simulink model "Final_Project_Pt5"  (R2024a)
settings: Solver=VariableStepAuto  StartTime=0.0  StopTime=tspan  FixedStep=10  RelTol=1e-3
values from neighbouring files (symbols this model uses):
  E_b_ECI_0 = C2EulerAngles(C_b_ECI_0)    [A421_FinalProject_Pt5.m]    (also in A421_FinalProject_Pt6.m; Final_Project_Part_3_disturbances.m; Final_Project_Part_3_disturbances_init_Template-1.m; Final_Project_Part_3_disturbances_init_Template.m)
  epsilon_b_ECI_0 = [-.2; .4; .2]    [A421_FinalProject_Pt6.m]    (also in hw5.m)
  J = [812.04 0 0; 0 545.37 0; 0 0 627.71]    [A421_FinalProject_Pt5.m]    (also in A421_FinalProject_Pt6.m; Final_Project_Part_3_disturbances_torques.m; Final_Project_Pt4.m; hw5.m = diag([1200, 2000, 2800]))
  JD_0 = 2460390    [A421_FinalProject_Pt5.m]    (also in A421_FinalProject_Pt6.m; Final_Project_Part_3_disturbances.m; Final_Project_Part_3_disturbances_init_Template-1.m; Final_Project_Part_3_disturbances_init_Template.m)
  Kd = J*2*zeta*wn*[1;1;1]    [A421_FinalProject_Pt5.m]    (also in A421_FinalProject_Pt6.m = J*2*zeta*wn; hw5.m = J*2*zeta*wn.*eye(3))
  Kp = 2*J*wn^2*[1;1;1]    [A421_FinalProject_Pt5.m]    (also in A421_FinalProject_Pt6.m = 2*J*wn^2.; hw5.m = 2*J*wn^2*eye(3))
  m_b = [0;0;-0.5]    [A421_FinalProject_Pt5.m]    (also in A421_FinalProject_Pt6.m; Final_Project_Pt4.m)
  q_b_ECI_0 = C2quat(C_b_ECI_0)    [A421_FinalProject_Pt5.m]    (also in A421_FinalProject_Pt6.m = [epsilon_b_ECI_0; sqrt(1-norm(epsilon_b_ECI_0)^2)]; Final_Project_Part_3_disturbances.m; Final_Project_Part_3_disturbances_init_Template-1.m; Final_Project_Part_3_disturbances_init_Template.m)
  q_C = [epsilon_C; sqrt(1-norm(epsilon_C)^2)]    [A421_FinalProject_Pt6.m]    (also in hw5.m)
  r_ECI_0 = rECI    [A421_FinalProject_Pt5.m]    (also in A421_FinalProject_Pt6.m; Final_Project_Pt4.m)
  sun_ECI = [1;0;0]    [A421_FinalProject_Pt5.m]    (also in A421_FinalProject_Pt6.m; Final_Project_Part_3_disturbances_torques.m; Final_Project_Pt4.m)
  surfaceProperties = [Areas_1 cps_1 normals_1; Areas_2 cps_2 normals_2; Areas_3 cps_3 normals_3; Areas_4 cps_4 normals_4]    [A421_FinalProject_Pt5.m]    (also in A421_FinalProject_Pt6.m; Final_Project_Part_3_disturbances.m = [Areas cps normals]; Final_Project_Part_3_disturbances_init_Template-1.m = [Areas cps normals]; Final_Project_Part_3_disturbances_init_Template.m = [Areas cps normals])
  T = [0;0;0]    [A421_FinalProject_Pt6.m]    (also in hw5.m; main.m)
  v_ECI_0 = vECI    [A421_FinalProject_Pt5.m]    (also in A421_FinalProject_Pt6.m; Final_Project_Pt4.m)
  w_b_ECI_0 = [0.001; -0.001; 0.002]    [A421_FinalProject_Pt5.m]    (also in A421_FinalProject_Pt6.m; Final_Project_Part_3_disturbances.m; Final_Project_Part_3_disturbances_init_Template-1.m; Final_Project_Part_3_disturbances_init_Template.m)
settings Model: Creator=emehiel  LastModifiedBy=Jacob
settings SolverCC: AlgebraicLoopSolver=TrustRegion
settings OptimizationCC: ReuseModelBlockBuffer=off
settings DebuggingCC: UnconnectedInputMsg=warning  UnconnectedOutputMsg=warning  UnconnectedLineMsg=warning
settings ModelReferenceCC: EnableRefExpFcnMdlSchedulingChecks=on
settings RTWCC: GPUComputeCapability=3.5

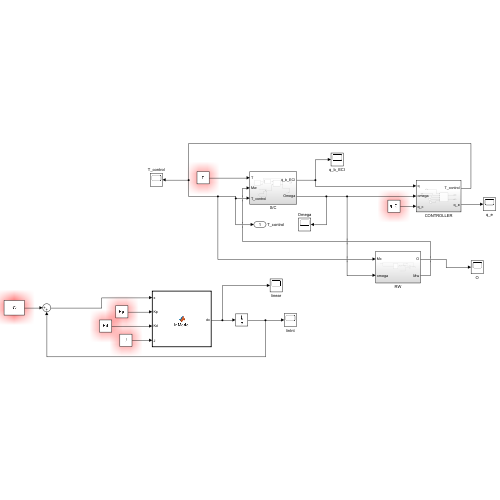
[thumbnail: Simulink's stored preview of the top-level diagram]
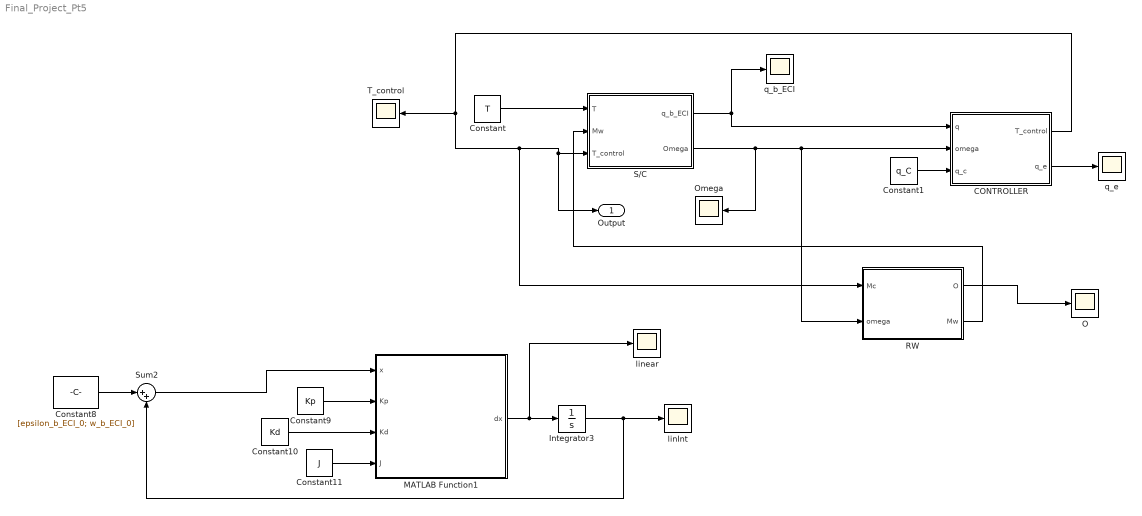
== system Final_Project_Pt5 ==
  CONTROLLER : Subsystem
  Constant : Constant  Value=T  VectorParams1D=off
  Constant1 : Constant  Value=q_C
  Constant10 : Constant  Value=Kd
  Constant11 : Constant  Value=J
  Constant8 : Constant  Value=[epsilon_b_ECI_0; w_b_ECI_0]
  Constant9 : Constant  Value=Kp
  Integrator3 : Integrator
  MATLAB Function1 : MATLAB Function  TreatAsAtomicUnit=on
  O : Scope
  Omega : Scope
  RW : Subsystem
  S/C : Subsystem
  Sum2 : Sum  Inputs=|++
  T_control : Scope
  linInt : Scope
  linear : Scope
  q_b_ECI : Scope
  q_e : Scope
  Output : Outport  SignalName=T_control
  wires:
  Constant/1 -> S/C/1(T)
  CONTROLLER/1(T_control) -> RW/1(Mc), Output/1, S/C/3(T_control), T_control/1
  S/C/2(Omega) -> RW/2(omega), CONTROLLER/2(omega), Omega/1
  CONTROLLER/2(q_e) -> q_e/1
  Constant1/1 -> CONTROLLER/3(q_c)
  Constant11/1 -> MATLAB Function1/4(J)
  Constant10/1 -> MATLAB Function1/3(Kd)
  Constant9/1 -> MATLAB Function1/2(Kp)
  MATLAB Function1/1(dx) -> linear/1, Integrator3/1
  Constant8/1 -> Sum2/1
  Sum2/1 -> MATLAB Function1/1(x)
  Integrator3/1 -> Sum2/2, linInt/1
  S/C/1(q_b_ECI) -> q_b_ECI/1, CONTROLLER/1(q)
  RW/1(O) -> O/1
  RW/2(Mw) -> S/C/2(Mw)

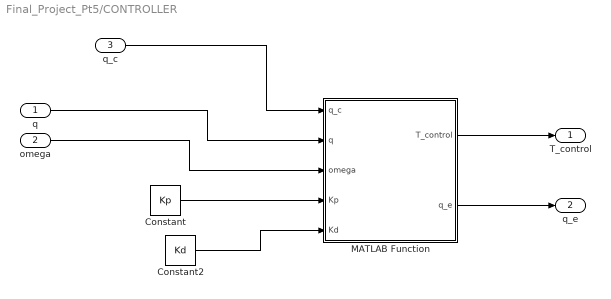
== system Final_Project_Pt5/CONTROLLER ==
  q : Inport
  omega : Inport  Port=2
  q_c : Inport  Port=3
  Constant : Constant  Value=Kp
  Constant2 : Constant  Value=Kd
  MATLAB Function : MATLAB Function  TreatAsAtomicUnit=on
  T_control : Outport
  q_e : Outport  Port=2
  wires:
  q/1 -> MATLAB Function/2(q)
  omega/1 -> MATLAB Function/3(omega)
  Constant/1 -> MATLAB Function/4(Kp)
  Constant2/1 -> MATLAB Function/5(Kd)
  MATLAB Function/2(q_e) -> q_e/1
  q_c/1 -> MATLAB Function/1(q_c)
  MATLAB Function/1(T_control) -> T_control/1

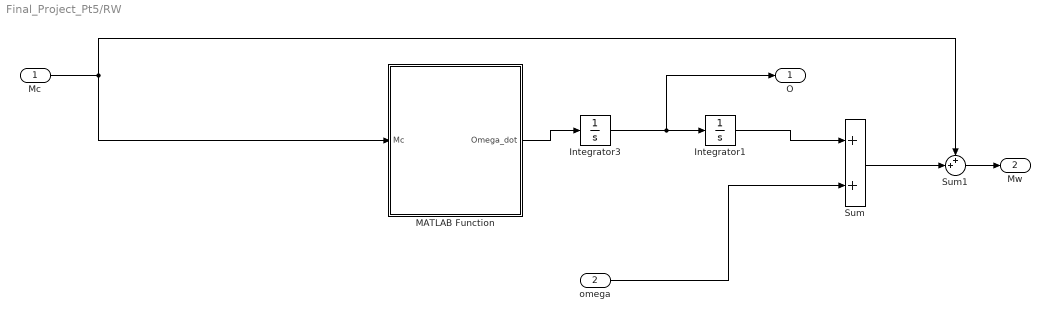
== system Final_Project_Pt5/RW ==
  Mc : Inport
  omega : Inport  Port=2
  Integrator1 : Integrator
  Integrator3 : Integrator
  MATLAB Function : MATLAB Function  TreatAsAtomicUnit=on
  Sum : Sum
  Sum1 : Sum  Inputs=++|
  O : Outport
  Mw : Outport  Port=2
  wires:
  omega/1 -> Sum/2
  Integrator3/1 -> Integrator1/1, O/1
  MATLAB Function/1(Omega_dot) -> Integrator3/1
  Integrator1/1 -> Sum/1
  Sum/1 -> Sum1/2
  Mc/1 -> MATLAB Function/1(Mc), Sum1/1
  Sum1/1 -> Mw/1

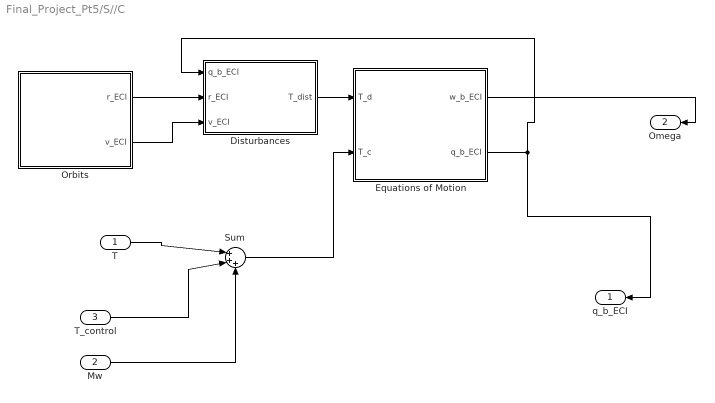
== system Final_Project_Pt5/S//C ==
  T : Inport
  Mw : Inport  Port=2
  T_control : Inport  Port=3
  Disturbances : Subsystem
  Equations of Motion : Subsystem
  Orbits : Subsystem
  Sum : Sum  Inputs=|+++
  q_b_ECI : Outport
  Omega : Outport  Port=2
  wires:
  T/1 -> Sum/1
  T_control/1 -> Sum/2
  Orbits/1(r_ECI) -> Disturbances/2(r_ECI)
  Disturbances/1(T_dist) -> Equations of Motion/1(T_d)
  Orbits/2(v_ECI) -> Disturbances/3(v_ECI)
  Equations of Motion/1(w_b_ECI) -> Omega/1
  Sum/1 -> Equations of Motion/2(T_c)
  Equations of Motion/2(q_b_ECI) -> Disturbances/1(q_b_ECI), q_b_ECI/1
  Mw/1 -> Sum/3

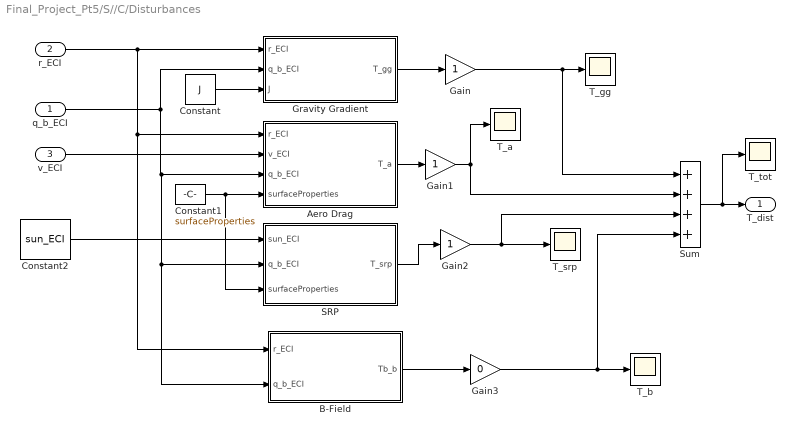
== system Final_Project_Pt5/S//C/Disturbances ==
  q_b_ECI : Inport
  r_ECI : Inport  Port=2
  v_ECI : Inport  Port=3
  Aero Drag : MATLAB Function  TreatAsAtomicUnit=on
  B-Field : Subsystem
  Constant : Constant  Value=J
  Constant1 : Constant  Value=surfaceProperties
  Constant2 : Constant  Value=sun_ECI
  Gain : Gain
  Gain1 : Gain
  Gain2 : Gain
  Gain3 : Gain  Gain=0
  Gravity Gradient : MATLAB Function  TreatAsAtomicUnit=on
  SRP : MATLAB Function  TreatAsAtomicUnit=on
  Sum : Sum  Inputs=++++
  T_a : Scope
  T_b : Scope
  T_gg : Scope
  T_srp : Scope
  T_tot : Scope
  T_dist : Outport
  wires:
  Sum/1 -> T_tot/1, T_dist/1
  Constant1/1 -> SRP/3(surfaceProperties), Aero Drag/4(surfaceProperties)
  v_ECI/1 -> Aero Drag/2(v_ECI)
  q_b_ECI/1 -> B-Field/2(q_b_ECI), SRP/2(q_b_ECI), Aero Drag/3(q_b_ECI), Gravity Gradient/2(q_b_ECI)
  Constant/1 -> Gravity Gradient/3(J)
  Constant2/1 -> SRP/1(sun_ECI)
  r_ECI/1 -> B-Field/1(r_ECI), Aero Drag/1(r_ECI), Gravity Gradient/1(r_ECI)
  Gain/1 -> Sum/1, T_gg/1
  Gain1/1 -> Sum/2, T_a/1
  Gain2/1 -> Sum/3, T_srp/1
  Gain3/1 -> T_b/1, Sum/4
  B-Field/1(Tb_b) -> Gain3/1
  Gravity Gradient/1(T_gg) -> Gain/1
  Aero Drag/1(T_a) -> Gain1/1
  SRP/1(T_srp) -> Gain2/1

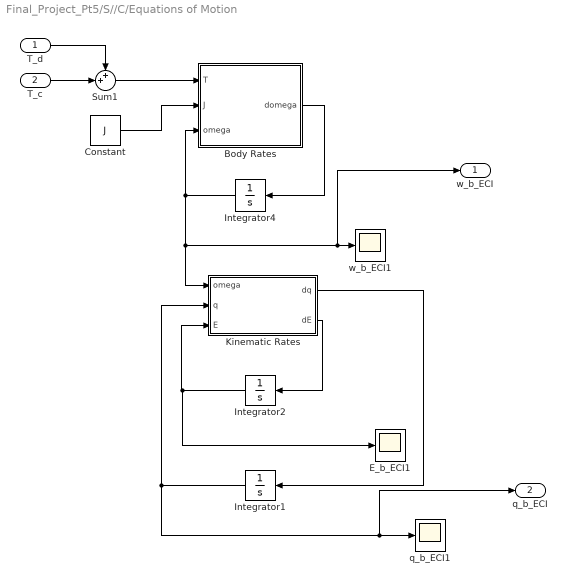
== system Final_Project_Pt5/S//C/Equations of Motion ==
  T_d : Inport
  T_c : Inport  Port=2
  Body Rates : MATLAB Function  TreatAsAtomicUnit=on
  Constant : Constant  Value=J
  E_b_ECI1 : Scope
  Integrator1 : Integrator  InitialCondition=q_b_ECI_0
  Integrator2 : Integrator  InitialCondition=E_b_ECI_0
  Integrator4 : Integrator  InitialCondition=w_b_ECI_0
  Kinematic Rates : MATLAB Function  TreatAsAtomicUnit=on
  Sum1 : Sum  Inputs=++|
  q_b_ECI1 : Scope
  w_b_ECI1 : Scope
  w_b_ECI : Outport  VectorParamsAs1DForOutWhenUnconnected=off
  q_b_ECI : Outport  Port=2  VectorParamsAs1DForOutWhenUnconnected=off
  wires:
  Integrator2/1 -> E_b_ECI1/1, Kinematic Rates/3(E)
  Sum1/1 -> Body Rates/1(T)
  Constant/1 -> Body Rates/2(J)
  T_d/1 -> Sum1/1
  T_c/1 -> Sum1/2
  Integrator1/1 -> q_b_ECI/1, q_b_ECI1/1, Kinematic Rates/2(q)
  Integrator4/1 -> Body Rates/3(omega), w_b_ECI/1, w_b_ECI1/1, Kinematic Rates/1(omega)
  Kinematic Rates/1(dq) -> Integrator1/1
  Kinematic Rates/2(dE) -> Integrator2/1
  Body Rates/1(domega) -> Integrator4/1

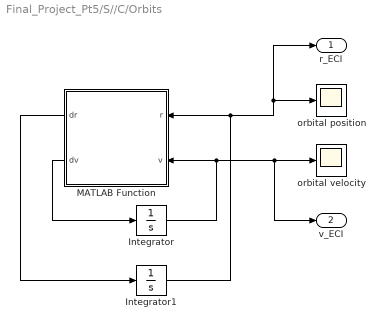
== system Final_Project_Pt5/S//C/Orbits ==
  Integrator : Integrator  InitialCondition=v_ECI_0
  Integrator1 : Integrator  InitialCondition=r_ECI_0
  MATLAB Function : MATLAB Function  TreatAsAtomicUnit=on
  orbital position : Scope
  orbital velocity : Scope
  r_ECI : Outport  VectorParamsAs1DForOutWhenUnconnected=off
  v_ECI : Outport  Port=2  VectorParamsAs1DForOutWhenUnconnected=off
  wires:
  Integrator/1 -> v_ECI/1, orbital velocity/1, MATLAB Function/2(v)
  Integrator1/1 -> r_ECI/1, orbital position/1, MATLAB Function/1(r)
  MATLAB Function/1(dr) -> Integrator1/1
  MATLAB Function/2(dv) -> Integrator/1

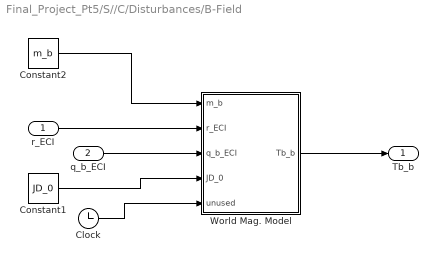
== system Final_Project_Pt5/S//C/Disturbances/B-Field ==
  r_ECI : Inport
  q_b_ECI : Inport  Port=2
  Clock : Clock
  Constant1 : Constant  Value=JD_0
  Constant2 : Constant  Value=m_b
  World Mag. Model : MATLAB Function  TreatAsAtomicUnit=on
  Tb_b : Outport
  wires:
  q_b_ECI/1 -> World Mag. Model/3(q_b_ECI)
  r_ECI/1 -> World Mag. Model/2(r_ECI)
  Clock/1 -> World Mag. Model/5(unused)
  Constant1/1 -> World Mag. Model/4(JD_0)
  Constant2/1 -> World Mag. Model/1(m_b)
  World Mag. Model/1(Tb_b) -> Tb_b/1

== matlab function Final_Project_Pt5/S//C/Orbits/MATLAB Function ==
  data: r input; dr output; v input; dv output
function [dr,dv] = orbitalDynamics(r, v)
muE = 398600; % km^3/s^2, Mu Earth
rx = r(1);
ry = r(2);
rz = r(3);
vx = v(1); 
vy = v(2); 
vz = v(3); 

r_norm = norm([rx ry rz]);

dvx = -muE*rx / r_norm^3;
dvy = -muE*ry / r_norm^3;
dvz = -muE*rz / r_norm^3;

dr = [vx; vy; vz];
dv = [dvx; dvy; dvz];

end

== matlab function Final_Project_Pt5/CONTROLLER/MATLAB Function ==
  data: q_c input; T_control output; q input; omega input; Kp input; Kd input; q_e output
function [T_control, q_e] = controller(q_c, q, omega, Kp, Kd)
%#codegen
% q_e = quatMult(q, quatConjugate(q_c));

% Quat conjugate rotated
q_c_conj = [q_c(1), -q_c(2), -q_c(3), -q_c(4)];
p0 = q_c_conj(1); p1 = q_c_conj(2); p2 = q_c_conj(3); p3 = q_c_conj(4);

% Quat multiplication
q0 = q(1,1); q1 = q(2); q2 = q(3); q3 = q(4);

q1 = q0 * p0 - q1 * p1 - q2 * p2 - q3 * p3;
q2 = q0 * p1 + q1 * p0 + q2 * p3 - q3 * p2;
q3 = q0 * p2 - q1 * p3 + q2 * p0 + q3 * p1;
q4 = q0 * p3 + q1 * p2 - q2 * p1 + q3 * p0;

q_e = [q1; q2; q3; q4];
disp(q_e)
% q_c

% T_control = -Kp*q_e(1:3,1) - Kd*omega;
T_control= 2*(-Kp*q_e(1:3) - Kd*omega);


end

== matlab function Final_Project_Pt5/S//C/Disturbances/Gravity Gradient ==
  data: r_ECI input; T_gg output; q_b_ECI input; J input
function T_gg = gg_torque(r_ECI, q_b_ECI, J)
% Function that calculates gravity gradient torque

% Constant(s)
muE = 398600;  % km^3/s^2, Mu earth
I = eye(3);    % Identity

% Unpack Quat
eps1 = q_b_ECI(1);
eps2 = q_b_ECI(2);
eps3 = q_b_ECI(3);
eps = [eps1; eps2; eps3];

eda = q_b_ECI(4);

% Solve
eps_cross = [0,  -eps3, eps2;
             eps3,  0, -eps1;
             -eps2, eps1, 0];

C_b_ECI = (2*eda^2 - 1)*I + 2*(eps*eps') - 2*eda*eps_cross; % rotation w/ quat

r_b = C_b_ECI*r_ECI;

r_b_cross = [0 -r_b(3,1) r_b(2,1);
           r_b(3,1) 0 -r_b(1,1);
           -r_b(2,1) r_b(1,1) 0];

T_gg = (3*muE)/(norm(r_ECI)^5)*r_b_cross*J*r_ECI;

end

== matlab function Final_Project_Pt5/MATLAB Function1 ==
  data: x input; Kp input; Kd input; J input; dx output
function dx = linModel(x, Kp, Kd, J)
    theta = x(1:3);  % Angular pos
    omega = x(4:6);  % Angular vel
    
    % PD Controller
    tau = -Kp *(theta -  [0; 0; 0]) - Kd*(omega - [0; 0; 0]);
    M = tau.*[2; 2; 2];
    
    alpha = J\(M- cross(omega, J*omega));

    dx = [omega; alpha];
end

== matlab function Final_Project_Pt5/S//C/Disturbances/Aero Drag ==
  data: r_ECI input; v_ECI input; T_a output; q_b_ECI input; surfaceProperties input
function T_a = aero_drag_torque(r_ECI, v_ECI, q_b_ECI, surfaceProperties) 
% Constants
C_d = 2.5;
r_earth = 6478 * 1000;
rho0 = 1.225;
I = eye(3);    % Identity

% Extract quaternion components
eps = q_b_ECI(1:3);
eda = q_b_ECI(4);

% Quaternion to rotation matrix
eps_cross = [0, -eps(3), eps(2);
             eps(3), 0, -eps(1);
            -eps(2), eps(1), 0];
C_b_ECI = (2 * eda^2 - 1) * I + 2 * (eps * eps') - 2 * eda * eps_cross;

s_ECI = [1;0;0];

% Convert velocity from ECI to body frame
v_b = C_b_ECI * v_ECI;
s_b = C_b_ECI * s_ECI;

% Calculate atmospheric density
rho = rho0 * exp(-(norm(r_ECI*1000) - r_earth) / 8500); 

% Initialize torque
T_a = [0; 0; 0];

% Iterate over surface properties
for i = 1:size(surfaceProperties, 1)
    % Extract surface properties
    S = surfaceProperties(i, 1);
    cp = surfaceProperties(i, 2:4)';
    normal = surfaceProperties(i, 5:7);  % Normal is now a row vector

    % Calculate relative velocity component normal to the surface
    A_wet = S*dot(s_b, normal);

    if A_wet > 0
        % Calculate drag force
        F_drag = -0.5 * rho * norm(v_b*1000)^2 * A_wet * C_d * v_b/norm(v_b);

        % Add torque contribution
        T_a = T_a + cross(cp, F_drag);
    end
end

end

== matlab function Final_Project_Pt5/RW/MATLAB Function ==
  data: Omega_dot output; Mc input
function Omega_dot  = RW(Mc)
%#codegen
Is = [Is1 0 0; 0 Is2 0; 0 0 Is3];

Omega_dot = Is\Mc;

end

== matlab function Final_Project_Pt5/S//C/Disturbances/B-Field/World Mag. Model ==
  data: m_b input; r_ECI input; q_b_ECI input; Tb_b output; JD_0 input; unused input
function Tb_b = WMM(m_b, r_ECI, q_b_ECI, JD_0, ~)
% Function of World Magn. Model

% DGRF 2020 (given)
a = 6371.2;      %km
g_11 = -1450.9;  %nT
h_11 = 4652.5;   %nT
g_10 = -29404.8; %nT
m_ECEF = a^3*[g_11; h_11; g_10];


I = eye(3);    % Identity

eps1 = q_b_ECI(1);
eps2 = q_b_ECI(2);
eps3 = q_b_ECI(3);
eps = [eps1; eps2; eps3];

eda = q_b_ECI(4);

eps_cross = [0,  -eps3, eps2;
             eps3,  0, -eps1;
             -eps2, eps1, 0];

C_b_ECI = (2*eda^2 - 1)*I + 2*(eps*eps') - 2*eda*eps_cross; % rotation w/ quat

% r_ECEF = eci2ecef_manual(JD_0, r_ECI);
T_UT1 = (JD_0 - 2451545.0)/36525; % Time in Julian centuries from J2000
GMST = mod(67310.54841 + (876600*3600 + 8640184.812866)*T_UT1 + 0.093104*T_UT1^2 - 6.2e-6*T_UT1^3, 86400) / 240; % in degrees
GMST = deg2rad(GMST); 

% Rotation matrix -ECI to ECEF
R_ECI2ECEF = [cos(GMST) sin(GMST) 0; -sin(GMST) cos(GMST) 0; 0 0 1];
r_ECEF = R_ECI2ECEF * r_ECI;


C_ECI_ECEF = r_ECI*r_ECEF';

% Solve
B_ECEF = (3*(m_ECEF'*r_ECEF)*r_ECEF - norm(r_ECEF)^2*m_ECEF)/(norm(r_ECEF))^5; % Mag. field vect in ECEF

B_ECI = C_ECI_ECEF*B_ECEF; 

B_b = C_b_ECI*B_ECI;

Tb_b = cross(m_b,B_b);

end

% function r_ECEF = eci2ecef_manual(JD, r_ECI)
% %     omega_earth = 7.2921159e-5; 
%     T_UT1 = (JD - 2451545.0)/36525; % Time in Julian centuries from J2000
%     GMST = mod(67310.54841 + (876600*3600 + 8640184.812866)*T_UT1 + 0.093104*T_UT1^2 - 6.2e-6*T_UT1^3, 86400) / 240; % in degrees
%     GMST = deg2rad(GMST); 
% 
%     % Rotation matrix -ECI to ECEF
%     R_ECI2ECEF = [cos(GMST) sin(GMST) 0; -sin(GMST) cos(GMST) 0; 0 0 1];
%     r_ECEF = R_ECI2ECEF * r_ECI;
% end

== matlab function Final_Project_Pt5/S//C/Disturbances/SRP ==
  data: sun_ECI input; T_srp output; q_b_ECI input; surfaceProperties input
function T_srp  = SRP_torque(sun_ECI, q_b_ECI, surfaceProperties)

p_sun = 4.5e-6; %N/m (given)

I = eye(3);

% Unpack Quat
eps1 = q_b_ECI(1);
eps2 = q_b_ECI(2);
eps3 = q_b_ECI(3);
eps = [eps1; eps2; eps3];

eda = q_b_ECI(4);

eps_cross = [0,  -eps3, eps2;
             eps3,  0, -eps1;
             -eps2, eps1, 0];

C_b_ECI = (2*eda^2 - 1)*I + 2*(eps*eps') - 2*eda*eps_cross; % rotation w/ quat

s_b = C_b_ECI*sun_ECI;
s_d = sun_ECI / norm(sun_ECI);

% Solve

% Initialize torque
T_srp = [0; 0; 0];

% Iterate over surface properties
for i = 1:size(surfaceProperties, 1)
    % Extract surface properties
    S = surfaceProperties(i, 1);
    cp = surfaceProperties(i, 2:4)';
    normal = surfaceProperties(i, 5:7);  % Normal is now a row vector

    % Calculate relative velocity component normal to the surface
    A_wet = S*dot(s_d, normal);

    if A_wet > 0
        % Add torque contribution
        T_srp = p_sun * A_wet * cross(s_b, s_d);
    end
end

end

== matlab function Final_Project_Pt5/S//C/Equations of Motion/Body Rates ==
  data: T input; J input; omega input; domega output
function domega = dynamics(T, J, omega)
%#codegen


% Compute the derivative of the angular velocity $\omega$ here
domega = J \ (T - cross(omega, J*omega));


end

== matlab function Final_Project_Pt5/S//C/Equations of Motion/Kinematic Rates ==
  data: omega input; q input; dq output; E input; dE output
function [dq,dE] = kinematics(omega, q, E)
%#codegen

I = eye(3); % Identity

% unpack quaternion
eps1 = q(1);
eps2 = q(2);
eps3 = q(3);
eps = [eps1; eps2; eps3];

eda = q(4);

% Compute the derivative of the quaternion components here
             
% Quaternion rates Eq.1.56
eps_cross = [0,  -eps3, eps2;
             eps3,  0, -eps1;
             -eps2, eps1, 0];

deps = 0.5*(eda*I + eps_cross)*omega;
deda = -0.5*eps'*omega;

dq = [deps; deda];

% Compute the derivative of the Euler Angle components here
            
% Euler rates
phi = E(1);
theta = E(2);
R = [1 sin(phi)*tan(theta) cos(phi)*tan(theta);
     0     cos(phi)           -sin(phi);
     0 sin(phi)*sec(theta) cos(phi)*sec(theta)];
    
dE = R*omega;


end
